simulink model "est_pos"  (R2020a)
settings: Solver=VariableStepAuto  StartTime=0.0  StopTime=simulation.stopTime  RelTol=1e-3
values from neighbouring files (symbols this model uses):
  L1 = 1    [estimate_position.m]
  L2 = -0.5    [estimate_position.m]
undefined symbols (not defined in the file or in its folder): DiscIntNeverNeededParam, servoModel, simulation
settings Model: Creator=FawadFarooq  LastModifiedBy=FawaD KhaN
settings DebuggingCC: SFMachineParentedDataDiag=error

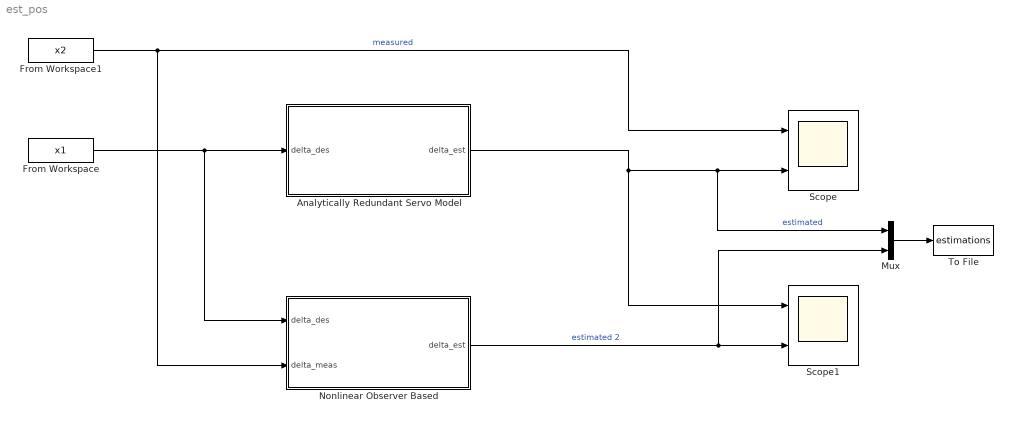
== system est_pos ==
  Analytically Redundant Servo Model : Subsystem
  From Workspace : FromWorkspace  VariableName=x1  SampleTime=1/simulation.Fs
  From Workspace1 : FromWorkspace  VariableName=x2  SampleTime=1/simulation.Fs
  Mux : Mux  Inputs=2
  Nonlinear Observer Based : Subsystem
  Scope : Scope  NumInputPorts=2
  Scope1 : Scope  NumInputPorts=2
  To File : ToFile  Filename=estimations  MatrixName=p_est
  wires:
  From Workspace/1 -> Analytically Redundant Servo Model/1(delta_des), Nonlinear Observer Based/1(delta_des)
  Analytically Redundant Servo Model/1(delta_est) -> Scope1/1, Mux/1, Scope/2  "estimated"
  From Workspace1/1 -> Nonlinear Observer Based/2(delta_meas), Scope/1  "measured"
  Nonlinear Observer Based/1(delta_est) -> Mux/2, Scope1/2  "estimated 2"
  Mux/1 -> To File/1

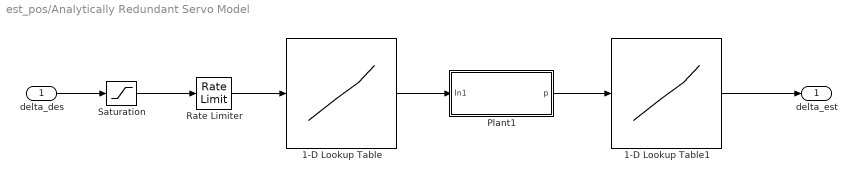
== system est_pos/Analytically Redundant Servo Model ==
  delta_des : Inport
  1-D Lookup Table : Lookup_n-D  NumberOfTableDimensions=1  BreakpointsForDimension1=[-30,-21,-11,0,14,20]  Table=[77.78,58.55,29.58,0,-37.48,-52.95]  InternalRulePriority=Speed  RndMeth=Simplest  InputSameDT=on
  1-D Lookup Table1 : Lookup_n-D  NumberOfTableDimensions=1  BreakpointsForDimension1=[-52.95, -37.48, 0.0, 29.58, 55.62, 77.78]  Table=[20.0, 14.0, 0.0, -11.0, -21.0, -30.0]  InternalRulePriority=Speed  RndMeth=Simplest  InputSameDT=on
  Plant1 : Subsystem
  Rate Limiter : RateLimiter  RisingSlewLimit=30  FallingSlewLimit=-30
  Saturation : Saturate  UpperLimit=15  LowerLimit=-30
  delta_est : Outport
  wires:
  1-D Lookup Table/1 -> Plant1/1(In1)
  Plant1/1(p) -> 1-D Lookup Table1/1
  delta_des/1 -> Saturation/1
  1-D Lookup Table1/1 -> delta_est/1
  Saturation/1 -> Rate Limiter/1
  Rate Limiter/1 -> 1-D Lookup Table/1

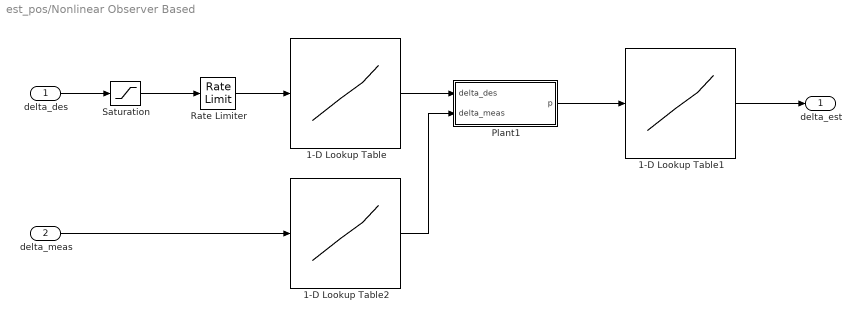
== system est_pos/Nonlinear Observer Based ==
  delta_des : Inport
  delta_meas : Inport  Port=2
  1-D Lookup Table : Lookup_n-D  NumberOfTableDimensions=1  BreakpointsForDimension1=[-30,-21,-11,0,14,20]  Table=[77.78,58.55,29.58,0,-37.48,-52.95]  InternalRulePriority=Speed  RndMeth=Simplest  InputSameDT=on
  1-D Lookup Table1 : Lookup_n-D  NumberOfTableDimensions=1  BreakpointsForDimension1=[-52.95, -37.48, 0.0, 29.58, 55.62, 77.78]  Table=[20.0, 14.0, 0.0, -11.0, -21.0, -30.0]  InternalRulePriority=Speed  RndMeth=Simplest  InputSameDT=on
  1-D Lookup Table2 : Lookup_n-D  NumberOfTableDimensions=1  BreakpointsForDimension1=[-30,-21,-11,0,14,20]  Table=[77.78,58.55,29.58,0,-37.48,-52.95]  InternalRulePriority=Speed  RndMeth=Simplest  InputSameDT=on
  Plant1 : Subsystem
  Rate Limiter : RateLimiter  RisingSlewLimit=30  FallingSlewLimit=-30
  Saturation : Saturate  UpperLimit=15  LowerLimit=-30
  delta_est : Outport
  wires:
  Rate Limiter/1 -> 1-D Lookup Table/1
  Saturation/1 -> Rate Limiter/1
  1-D Lookup Table1/1 -> delta_est/1
  delta_des/1 -> Saturation/1
  Plant1/1(p) -> 1-D Lookup Table1/1
  1-D Lookup Table/1 -> Plant1/1(delta_des)
  delta_meas/1 -> 1-D Lookup Table2/1
  1-D Lookup Table2/1 -> Plant1/2(delta_meas)

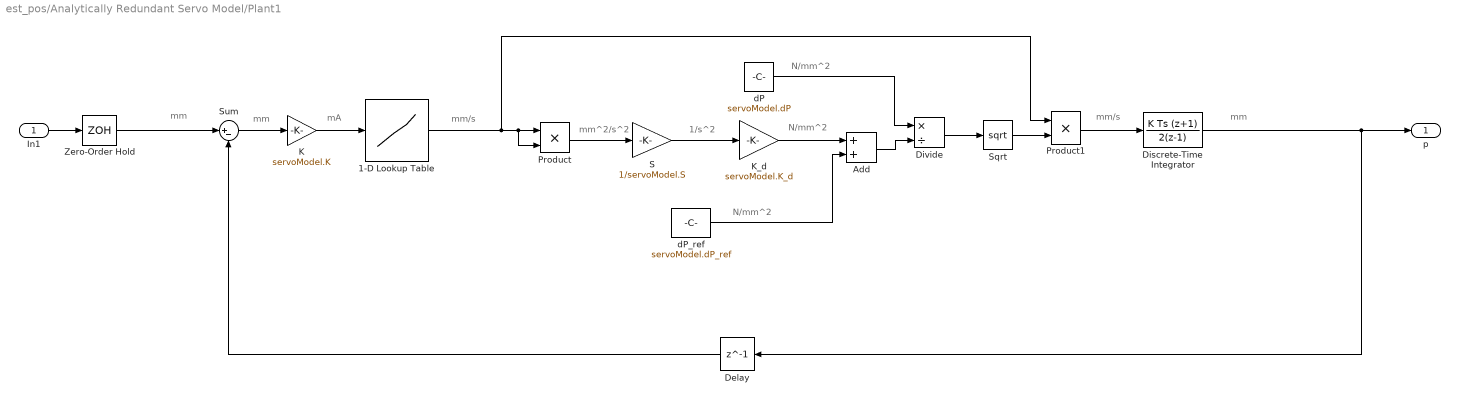
== system est_pos/Analytically Redundant Servo Model/Plant1 ==
  note: mm
  note: mm
  note: mm/s
  note: N/mm^2
  note: 1/s^2
  note: mm^2/s^2
  note: mm/s
  note: mA
  note: mm
  note: N/mm^2
  note: N/mm^2
  In1 : Inport
  1-D Lookup Table : Lookup_n-D  NumberOfTableDimensions=1  BreakpointsForDimension1=[-11,-8.45,-2.3,0,2.3,8.45,11]  Table=[-250,-250,-32,0,32,250,250]  InternalRulePriority=Speed  RndMeth=Simplest  InputSameDT=on
  Add : Sum
  Delay : Delay  DelayLength=1  SampleTime=1/simulation.Fs
  Discrete-Time Integrator : DiscreteIntegrator  IntegratorMethod=Integration: Trapezoidal  SampleTime=1/simulation.Fs  ICPrevOutput=DiscIntNeverNeededParam  ICPrevScaledInput=DiscIntNeverNeededParam
  Divide : Product  Inputs=*/
  K : Gain  Gain=servoModel.K
  K_d : Gain  Gain=servoModel.K_d
  Product : Product
  Product1 : Product
  S : Gain  Gain=1/servoModel.S
  Sqrt : Sqrt  SaturateOnIntegerOverflow=on
  Sum : Sum  Inputs=|+-
  Zero-Order Hold : ZeroOrderHold  SampleTime=1/simulation.Fs
  dP : Constant  Value=servoModel.dP
  dP_ref : Constant  Value=servoModel.dP_ref
  p : Outport
  wires:
  Product1/1 -> Discrete-Time Integrator/1
  In1/1 -> Zero-Order Hold/1
  Sum/1 -> K/1
  K/1 -> 1-D Lookup Table/1
  Product/1 -> S/1
  dP_ref/1 -> Add/2
  K_d/1 -> Add/1
  Add/1 -> Divide/2
  S/1 -> K_d/1
  Divide/1 -> Sqrt/1
  Sqrt/1 -> Product1/2
  dP/1 -> Divide/1
  1-D Lookup Table/1 -> Product/1, Product/2, Product1/1
  Zero-Order Hold/1 -> Sum/1
  Discrete-Time Integrator/1 -> p/1, Delay/1
  Delay/1 -> Sum/2

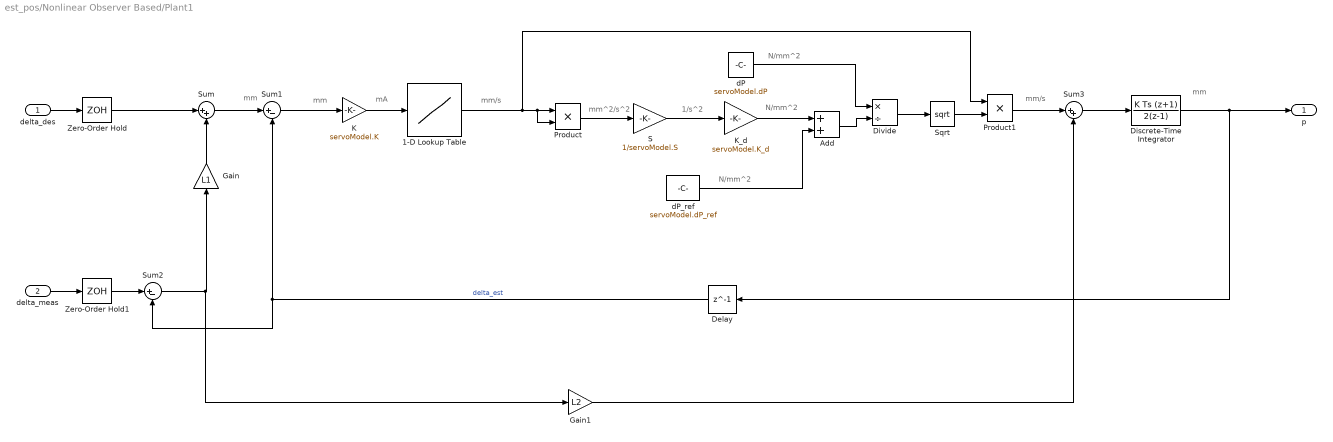
== system est_pos/Nonlinear Observer Based/Plant1 ==
  note: N/mm^2
  note: N/mm^2
  note: mm
  note: mA
  note: mm/s
  note: mm^2/s^2
  note: 1/s^2
  note: N/mm^2
  note: mm/s
  note: mm
  note: mm
  delta_des : Inport
  delta_meas : Inport  Port=2
  1-D Lookup Table : Lookup_n-D  NumberOfTableDimensions=1  BreakpointsForDimension1=[-11,-8.45,-2.3,0,2.3,8.45,11]  Table=[-250,-250,-32,0,32,250,250]  InternalRulePriority=Speed  RndMeth=Simplest  InputSameDT=on
  Add : Sum
  Delay : Delay  DelayLength=1  SampleTime=1/simulation.Fs
  Discrete-Time Integrator : DiscreteIntegrator  IntegratorMethod=Integration: Trapezoidal  SampleTime=1/simulation.Fs  ICPrevOutput=DiscIntNeverNeededParam  ICPrevScaledInput=DiscIntNeverNeededParam
  Divide : Product  Inputs=*/
  Gain : Gain  Gain=L1
  Gain1 : Gain  Gain=L2
  K : Gain  Gain=servoModel.K
  K_d : Gain  Gain=servoModel.K_d
  Product : Product
  Product1 : Product
  S : Gain  Gain=1/servoModel.S
  Sqrt : Sqrt  SaturateOnIntegerOverflow=on
  Sum : Sum  Inputs=|++
  Sum1 : Sum  Inputs=|+-
  Sum2 : Sum  Inputs=|+-
  Sum3 : Sum  Inputs=|++
  Zero-Order Hold : ZeroOrderHold  SampleTime=1/simulation.Fs
  Zero-Order Hold1 : ZeroOrderHold  SampleTime=1/simulation.Fs
  dP : Constant  Value=servoModel.dP
  dP_ref : Constant  Value=servoModel.dP_ref
  p : Outport
  wires:
  Delay/1 -> Sum2/2, Sum1/2  "delta_est"
  Discrete-Time Integrator/1 -> p/1, Delay/1
  1-D Lookup Table/1 -> Product1/1, Product/2, Product/1
  dP/1 -> Divide/1
  Sqrt/1 -> Product1/2
  Divide/1 -> Sqrt/1
  S/1 -> K_d/1
  Add/1 -> Divide/2
  K_d/1 -> Add/1
  dP_ref/1 -> Add/2
  Product/1 -> S/1
  K/1 -> 1-D Lookup Table/1
  Sum1/1 -> K/1
  delta_des/1 -> Zero-Order Hold/1
  delta_meas/1 -> Zero-Order Hold1/1
  Zero-Order Hold1/1 -> Sum2/1
  Zero-Order Hold/1 -> Sum/1
  Sum/1 -> Sum1/1
  Gain/1 -> Sum/2
  Product1/1 -> Sum3/1
  Sum3/1 -> Discrete-Time Integrator/1
  Sum2/1 -> Gain1/1, Gain/1
  Gain1/1 -> Sum3/2
